simulink model "MSP_CurrentControl"  (R2018a)
settings: Solver=ode15s  StartTime=0.0  StopTime=1  RelTol=1e-3
values from neighbouring files (symbols this model uses):
  Kd = 0    [init.m]
  Ki = 63    [init.m]
  Kp = 6.3    [init.m]
  L = 1e-1    (= 0.1)    [init.m]
  n_levels = 9    [init.m]
  R = 90    [init.m]
  reference_frequency_hz = 100    [init.m]
  Ts = 1e-4    (= 0.0001)    [init.m]
  Vdc = 1    [init.m]
undefined symbols (not defined in the file or in its folder): G, serial
libraries: elec_lib x63, nesl_utility x52, powerlib x41, fl_lib x40, powerlib_meascontrol x4, simulink x3, instrumentlib x3
(part 2 of 2)

== matlab function MSP_CurrentControl/MATLAB Function1 ==
  data: u input; y output
function y = BridgeToGateSignalConversion(u)
if (u == 1)
    y = [1;0];
elseif (u==0)
    y = [1;1];
elseif (u==-1)
    y = [0;1];
else 
    y = [0;0];
end
end

== matlab function MSP_CurrentControl/MATLAB Function ==
  data: u input; y output
function y = BridgeToGateSignalConversion(u)
if (u == 1)
    y = [1;0];
elseif (u==0)
    y = [1;1];
elseif (u==-1)
    y = [0;1];
else 
    y = [0;0];
end
end

== matlab function MSP_CurrentControl/MATLAB Function2 ==
  data: u input; y output
function y = BridgeToGateSignalConversion(u)
if (u == 1)
    y = [1;0];
elseif (u==0)
    y = [1;1];
elseif (u==-1)
    y = [0;1];
else 
    y = [0;0];
end
end

== matlab function MSP_CurrentControl/MATLAB Function3 ==
  data: u input; y output
function y = BridgeToGateSignalConversion(u)
if (u == 1)
    y = [1;0];
elseif (u==0)
    y = [1;1];
elseif (u==-1)
    y = [0;1];
else 
    y = [0;0];
end
end

== matlab function MSP_CurrentControl/MATLAB Function4 ==
  data: u input; y output
function y = BridgeToGateSignalConversion(u)
if (u == 1)
    y = [1;0];
elseif (u==0)
    y = [1;1];
elseif (u==-1)
    y = [0;1];
else 
    y = [0;0];
end
end

== matlab function MSP_CurrentControl/MATLAB Function5 ==
  data: u input; y output
function y = BridgeToGateSignalConversion(u)
if (u == 1)
    y = [1;0];
elseif (u==0)
    y = [1;1];
elseif (u==-1)
    y = [0;1];
else 
    y = [0;0];
end
end

== matlab function MSP_CurrentControl/MATLAB Function6 ==
  data: u input; y output
function y = BridgeToGateSignalConversion(u)
if (u == 1)
    y = [1;0];
elseif (u==0)
    y = [1;1];
elseif (u==-1)
    y = [0;1];
else 
    y = [0;0];
end
end

== matlab function MSP_CurrentControl/MATLAB Function7 ==
  data: u input; y output
function y = BridgeToGateSignalConversion(u)
if (u == 1)
    y = [1;0];
elseif (u==0)
    y = [1;1];
elseif (u==-1)
    y = [0;1];
else 
    y = [0;0];
end
end

== matlab function MSP_CurrentControl/MATLAB Function8 ==
  data: u input; y output
function y = BridgeToGateSignalConversion(u)
if (u == 1)
    y = [1;0];
elseif (u==0)
    y = [1;1];
elseif (u==-1)
    y = [0;1];
else 
    y = [0;0];
end
end

== matlab function MSP_CurrentControl/MATLAB Function10 ==
  data: Dout output; D input
function Dout = DutyCycleConversion(D)
     D = double(D);
     Da = D(1:3,1);
     Db = D(4:6,1);
     Dc = D(7:9,1);
     Dout = [Da';Db';Dc'];
end

== matlab function MSP_CurrentControl/MATLAB Function11 ==
  data: V input; ControlSignals output
function ControlSignals = ControlSignalGenerator(V)
    ControlSignals = zeros(3,1);
    if (V==-13)
        ControlSignals = [-1;-1;-1];
    elseif (V==-12)
        ControlSignals = [-1;-1;0];
    elseif (V==-11)
        ControlSignals = [-1;-1;1];
    elseif (V==-10)
        ControlSignals = [-1;0;-1];
    elseif (V==-9)
        ControlSignals = [-1;0;0];
    elseif (V==-8)
        ControlSignals = [-1;0;1];    
    elseif (V==-7)
        ControlSignals = [-1;1;-1];
    elseif (V==-6)
        ControlSignals = [-1;1;0];
    elseif (V==-5)
        ControlSignals = [-1;1;1];
    elseif (V==-4)
        ControlSignals = [0;-1;-1];
    elseif (V==-3)
        ControlSignals = [0;-1;0];
    elseif (V==-2)
        ControlSignals = [0;-1;1];    
    elseif (V==-1)
        ControlSignals = [0;0;-1];
    elseif (V==0)
        ControlSignals = [0;0;0];
    elseif (V==1)
        ControlSignals = [0;0;1];
    elseif (V==2)
        ControlSignals = [0;1;-1];
    elseif (V==3)
        ControlSignals = [0;1;0];
    elseif (V==4)
        ControlSignals = [0;1;1];
    elseif (V==5)
        ControlSignals = [1;-1;-1];
    elseif (V==6)
        ControlSignals = [1;-1;0];
    elseif (V==7)
        ControlSignals = [1;-1;1];
    elseif (V==8)
        ControlSignals = [1;0;-1];
    elseif (V==9)
        ControlSignals = [1;0;0];
    elseif (V==10)
        ControlSignals = [1;0;1];
    elseif (V==11)
        ControlSignals = [1;1;-1];
    elseif (V==12)
        ControlSignals = [1;1;0];    
    elseif (V==13)
        ControlSignals = [1;1;1];
end

== matlab function MSP_CurrentControl/MATLAB Function12 ==
  data: V input; ControlSignals output
function ControlSignals = ControlSignalGenerator(V)
    ControlSignals = zeros(3,1);
    if (V==-13)
        ControlSignals = [-1;-1;-1];
    elseif (V==-12)
        ControlSignals = [-1;-1;0];
    elseif (V==-11)
        ControlSignals = [-1;-1;1];
    elseif (V==-10)
        ControlSignals = [-1;0;-1];
    elseif (V==-9)
        ControlSignals = [-1;0;0];
    elseif (V==-8)
        ControlSignals = [-1;0;1];    
    elseif (V==-7)
        ControlSignals = [-1;1;-1];
    elseif (V==-6)
        ControlSignals = [-1;1;0];
    elseif (V==-5)
        ControlSignals = [-1;1;1];
    elseif (V==-4)
        ControlSignals = [0;-1;-1];
    elseif (V==-3)
        ControlSignals = [0;-1;0];
    elseif (V==-2)
        ControlSignals = [0;-1;1];    
    elseif (V==-1)
        ControlSignals = [0;0;-1];
    elseif (V==0)
        ControlSignals = [0;0;0];
    elseif (V==1)
        ControlSignals = [0;0;1];
    elseif (V==2)
        ControlSignals = [0;1;-1];
    elseif (V==3)
        ControlSignals = [0;1;0];
    elseif (V==4)
        ControlSignals = [0;1;1];
    elseif (V==5)
        ControlSignals = [1;-1;-1];
    elseif (V==6)
        ControlSignals = [1;-1;0];
    elseif (V==7)
        ControlSignals = [1;-1;1];
    elseif (V==8)
        ControlSignals = [1;0;-1];
    elseif (V==9)
        ControlSignals = [1;0;0];
    elseif (V==10)
        ControlSignals = [1;0;1];
    elseif (V==11)
        ControlSignals = [1;1;-1];
    elseif (V==12)
        ControlSignals = [1;1;0];    
    elseif (V==13)
        ControlSignals = [1;1;1];
end

== matlab function MSP_CurrentControl/MATLAB Function13 ==
  data: V input; ControlSignals output
function ControlSignals = ControlSignalGenerator(V)
    ControlSignals = zeros(3,1);
    if (V==-13)
        ControlSignals = [-1;-1;-1];
    elseif (V==-12)
        ControlSignals = [-1;-1;0];
    elseif (V==-11)
        ControlSignals = [-1;-1;1];
    elseif (V==-10)
        ControlSignals = [-1;0;-1];
    elseif (V==-9)
        ControlSignals = [-1;0;0];
    elseif (V==-8)
        ControlSignals = [-1;0;1];    
    elseif (V==-7)
        ControlSignals = [-1;1;-1];
    elseif (V==-6)
        ControlSignals = [-1;1;0];
    elseif (V==-5)
        ControlSignals = [-1;1;1];
    elseif (V==-4)
        ControlSignals = [0;-1;-1];
    elseif (V==-3)
        ControlSignals = [0;-1;0];
    elseif (V==-2)
        ControlSignals = [0;-1;1];    
    elseif (V==-1)
        ControlSignals = [0;0;-1];
    elseif (V==0)
        ControlSignals = [0;0;0];
    elseif (V==1)
        ControlSignals = [0;0;1];
    elseif (V==2)
        ControlSignals = [0;1;-1];
    elseif (V==3)
        ControlSignals = [0;1;0];
    elseif (V==4)
        ControlSignals = [0;1;1];
    elseif (V==5)
        ControlSignals = [1;-1;-1];
    elseif (V==6)
        ControlSignals = [1;-1;0];
    elseif (V==7)
        ControlSignals = [1;-1;1];
    elseif (V==8)
        ControlSignals = [1;0;-1];
    elseif (V==9)
        ControlSignals = [1;0;0];
    elseif (V==10)
        ControlSignals = [1;0;1];
    elseif (V==11)
        ControlSignals = [1;1;-1];
    elseif (V==12)
        ControlSignals = [1;1;0];    
    elseif (V==13)
        ControlSignals = [1;1;1];
end

== matlab function MSP_CurrentControl/MATLAB Function14 ==
  data: u input; y output
function y = BridgeToGateSignalConversion(u)
if (u == 1)
    y = [1;0];
elseif (u==0)
    y = [1;1];
elseif (u==-1)
    y = [0;1];
else 
    y = [0;0];
end
end

== matlab function MSP_CurrentControl/MATLAB Function15 ==
  data: u input; y output
function y = BridgeToGateSignalConversion(u)
if (u == 1)
    y = [1;0];
elseif (u==0)
    y = [1;1];
elseif (u==-1)
    y = [0;1];
else 
    y = [0;0];
end
end

== matlab function MSP_CurrentControl/MATLAB Function16 ==
  data: u input; y output
function y = BridgeToGateSignalConversion(u)
if (u == 1)
    y = [1;0];
elseif (u==0)
    y = [1;1];
elseif (u==-1)
    y = [0;1];
else 
    y = [0;0];
end
end

== matlab function MSP_CurrentControl/MATLAB Function17 ==
  data: u input; y output
function y = BridgeToGateSignalConversion(u)
if (u == 1)
    y = [1;0];
elseif (u==0)
    y = [1;1];
elseif (u==-1)
    y = [0;1];
else 
    y = [0;0];
end
end

== matlab function MSP_CurrentControl/MATLAB Function18 ==
  data: u input; y output
function y = BridgeToGateSignalConversion(u)
if (u == 1)
    y = [1;0];
elseif (u==0)
    y = [1;1];
elseif (u==-1)
    y = [0;1];
else 
    y = [0;0];
end
end

== matlab function MSP_CurrentControl/MATLAB Function19 ==
  data: u input; y output
function y = BridgeToGateSignalConversion(u)
if (u == 1)
    y = [1;0];
elseif (u==0)
    y = [1;1];
elseif (u==-1)
    y = [0;1];
else 
    y = [0;0];
end
end

== matlab function MSP_CurrentControl/MATLAB Function20 ==
  data: u input; y output
function y = BridgeToGateSignalConversion(u)
if (u == 1)
    y = [1;0];
elseif (u==0)
    y = [1;1];
elseif (u==-1)
    y = [0;1];
else 
    y = [0;0];
end
end

== matlab function MSP_CurrentControl/MATLAB Function21 ==
  data: u input; y output
function y = BridgeToGateSignalConversion(u)
if (u == 1)
    y = [1;0];
elseif (u==0)
    y = [1;1];
elseif (u==-1)
    y = [0;1];
else 
    y = [0;0];
end
end

== matlab function MSP_CurrentControl/MATLAB Function22 ==
  data: u input; y output
function y = BridgeToGateSignalConversion(u)
if (u == 1)
    y = [1;0];
elseif (u==0)
    y = [1;1];
elseif (u==-1)
    y = [0;1];
else 
    y = [0;0];
end
end

== matlab function MSP_CurrentControl/MATLAB Function23 ==
  data: Ia input; node_indices output; Ib input; Ic input; Vdc input; n_levels input
function node_indices = FindBoundingNodeIndices(Ia, Ib, Ic, Vdc, n_levels)

    % Perform the gh-transform
    g = 1 / (3 * Vdc) * (2 * Ia - Ib - Ic);
    h = 1 / (3 * Vdc) * (-1 * Ia + 2 * Ib - Ic);
    
    nearest_nodes = repmat(struct('g', 0, 'h', 0), 4, 1);
    
    nearest_nodes(1).g = ceil(g);
    nearest_nodes(1).h = floor(h);
    
    nearest_nodes(2).g = floor(g);
    nearest_nodes(2).h = ceil(h);
    
    nearest_nodes(3).g = ceil(g);
    nearest_nodes(3).h = ceil(h);
    
    nearest_nodes(4).g = floor(g);
    nearest_nodes(4).h = floor(h);
    
    distances = zeros(4, 1);
    
    for i=1:4
       distances(i) =  abs(nearest_nodes(i).g - g) + abs(nearest_nodes(i).h - h);
    end
    
    % Now find minimum
    [min_value, min_index] = min(distances);
    
    k = 0;
    n = n_levels;
    nearest = nearest_nodes(min_index);
    while (true) 
        if (k >= 0 && k - nearest.g >= 0 && k - nearest.g - nearest.h >= 0 && k <= n - 1 && k - nearest.g <= n - 1 && k - nearest.g - nearest.h <= n - 1) 
            break
        end
        if (k >= n_levels) 
            break
        end
        k = k + 1;
    end
    
    a_phase_index = k;
    b_phase_index = k - nearest.g;
    c_phase_index = k - nearest.g - nearest.h;
    
    if (a_phase_index >= n)
        a_phase_index = n - 1;
    end
    
    if (a_phase_index < 0)
        a_phase_index = 0;
    end
    
    if (b_phase_index >= n)
        b_phase_index = n - 1;
    end
    
    if (b_phase_index < 0)
        b_phase_index = 0;
    end
    
    if (c_phase_index >= n)
        c_phase_index = n - 1;
    end
    
    if (c_phase_index < 0)
        c_phase_index = 0;
    end
    
   
    node_indices = [a_phase_index, b_phase_index, c_phase_index] - 4;
end

== matlab function MSP_CurrentControl/MATLAB Function24 ==
  data: Va input; Van output; Vb input; Vc input; Vbn output; Vcn output
function [Van,Vbn,Vcn] = BridgeToGateSignalConversion(Va,Vb,Vc)
   Van = 1/3*(2*Va - Vb - Vc);
   Vbn = 1/3*(-Va + 2*Vb - Vc);
   Vcn = 1/3*(-Va - Vb + 2*Vc);
end
